simulink model "cic_filter_test"  (Simulink 7.4)
settings: Solver=ode45  StartTime=0.0  StopTime=100000  RelTol=1e-3
libraries: xbsIndex_r4 x178
(part 1 of 3)
settings Model: Creator=hong  LastModifiedBy=hong

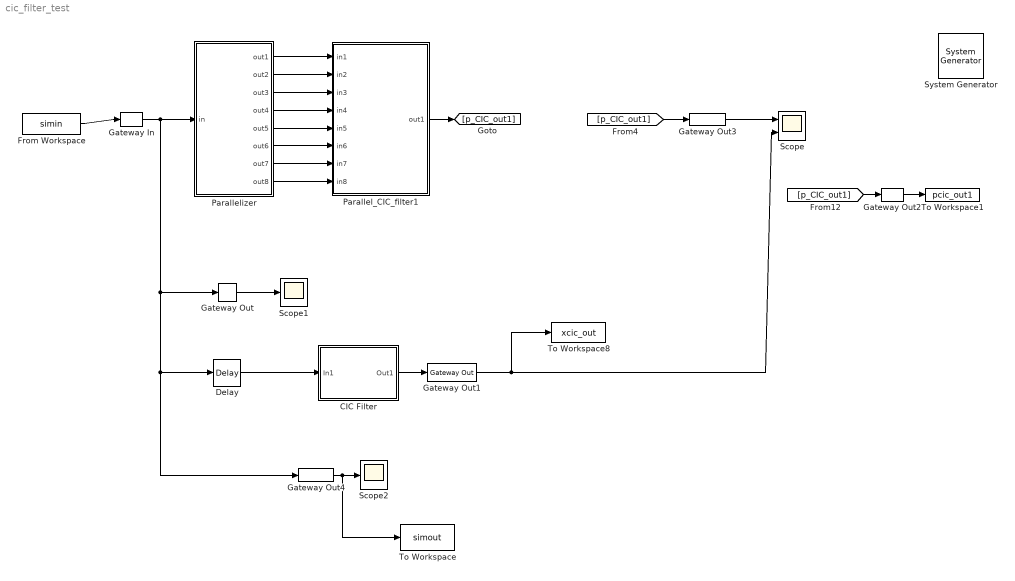
== system cic_filter_test ==
  " System Generator" : xbsIndex_r4/ System Generator  Tag=genX  SystemSampleTime=-1  xilinxfamily=virtex6  part=xc6vsx315t  speed=-3  package=ff1156  synthesis_tool=XST  clock_wrapper=Clock Enables  directory=./netlist  testbench=off  simulink_period=1  sysclk_period=10  dcm_input_clock_period=10  incr_netlist=off  trim_vbits=Everywhere in SubSystem  dbl_ovrd=According to Block Masks  core_generation=According to Block Masks  run_coregen=off  deprecated_control=off  eval_field=0  block_type=sysgen
      settings: block_version=11.4
  CIC Filter : Subsystem  mask(CIC Filter){input_bitwidth=8, input_binpt=7, filter_type=Decimator, rate_change=128, stages=3, m=1, pipeline=on}
      mask prompts: input_bitwidth "Input Bit Width"; input_binpt "Input Binary Point"; filter_type "Filter Type"; rate_change "Sample Rate Change"; stages "Number of Stages"; m "Differential Delay"; pipeline "Pipeline Differentiators"
      mask help: Cascaded Integrated Comb (CIC) Filter
      mask init:
      | % CIC Single Channel v1.0
      | % Set Block Logo
      | sav_gcb=gcb;
      | [bg,fg] = xlcmap('XBlock',0);
      | iPos = get_param(sav_gcb,'Position');
      | iWidth=iPos(3)-iPos(1); iHeight=iPos(4)-iPos(2);
      | iCx=iWidth/2;
      | iCy=iHeight/2;
      | [logoX, logoY] = xlogo(iPos);
      | 
      | % Determine previous filter type and number of stages
      | prev_stages_list = find_system(sav_gcb, 'lookUnderMasks', 'all', 'FollowLinks', 'on', 'Regexp', 'on', 'Name', '^Integrator*'); %this is a cell array
      | prev_stages = length(prev_stages_list);
      | 
      | prev_filter_list = find_system(sav_gcb, 'lookUnderMasks', 'all', 'FollowLinks', 'on', 'Regexp', 'on', 'Name', '^Up Sample*'); %this is a cell array
      | if (isempty(prev_filter_list))
      |     prev_filter_list = find_system(sav_gcb, 'lookUnderMasks', 'all', 'FollowLinks', 'on', 'Regexp', 'on', 'Name', '^Down Sample*'); %this is a cell array
      |     if (isempty(prev_filter_list))
      |         errordlg('Previous Filter Type could not be determined')
      |     else
      |         prev_filter_type = 2;
      |     end
      | else
      |     prev_filter_type = 1;
      | end
      |   
      |   
      | % Print label on the block
      | if(filter_type == 2)
      |    cic_str = sprintf('%d-Stage\n CIC\n%d:1 Decimator',stages, rate_change);
      | else
      |    cic_str = sprintf('%d-Stage\n CIC\n1:%d Interpolator',stages, rate_change);	
      | end
      | 
      | % Make sure the entered values for stages and channels are positive integers
      | nstages = round(sum(abs(stages)));
      | 
      | % issue an error if the number of stages entered is zero
      | if (nstages == 0)
      | 	nstages = prev_stages;
      | 	errordlg('Number of Stages must be more than zero')
      | end
      | 
      | if (nstages == prev_stages) & (filter_type == prev_filter_type)
      |     return
      | end
      | 
      | if(filter_type == 2) % Decimator
      |    if (prev_filter_type == 1) % was interpolator so turn to decimator
      |        for i= 2:prev_stages,
      | 	      delete_line(sav_gcb, ['Integrator' int2str(i-1) '/' int2str(1)], ['Integrator' int2str(i) '/' int2str(1)]);
      | 	      delete_line(sav_gcb, ['Differentiator' int2str(i-1) '/' int2str(1)], ['Differentiator' int2str(i) '/' int2str(1)]);
      |        end
      | 
      |        % disconnect the last blocks in the two sections
      |        delete_line(sav_gcb, ['Differentiator' int2str(prev_stages) '/' int2str(1)], ['Up Sample/1']);
      |        delete_line(sav_gcb, ['Integrator' int2str(prev_stages) '/' int2str(1)], 'Out1/1');
      | 	
      | 	   % delete the line from the Up sampler to the Integrator
      | 	   delete_line(sav_gcb, 'Up Sample/1', 'Integrator1/1'); 
      | 	   delete_line(sav_gcb, 'In1/1', 'Differentiator1/1'); 
      | 	   
      | 	   % Delete the Up Sampler and then replace with an Down Sampler
      | 	   pup = get_param([sav_gcb '/Up Sample'], 'position');
      | 	   delete_block([sav_gcb '/Up Sample']);
      | 	   load_system('xbsIndex_r4');
      | 	   add_block('xbsIndex_r4/Down Sample', [sav_gcb '/Down Sample'], 'sample_ratio', 'rate_change','sample_phase', 'First Value of Frame', 'position', [pup(1), pup(2), pup(3),pup(4)]);
      | 	   
      | 	   % Switch the Integrators and Decimators around
      | 	   for i=1:prev_stages,
      | 		   tempi = get_param([sav_gcb '/Integrator' int2str(i)], 'position');
      | 	       tempd = get_param([sav_gcb '/Differentiator' int2str(i)], 'position');
      | 		   set_param([sav_gcb '/Differentiator' int2str(i)], 'position', [tempi(1), tempi(2), tempi(3), tempi(4)], 'output_bitwidth', 'ceil(stages*log2(rate_change*m) + input_bitwidth)');
      | 		   set_param([sav_gcb '/Integrator' int2str(i)], 'position', [tempd(1), tempd(2), tempd(3), tempd(4)]);
      | 	   end
      | 	   	   	
      | 	   % add back in the lines
      |        add_line(sav_gcb, 'In1/1', 'Integrator1/1', 'autorouting', 'on');
      | 	   add_line(sav_gcb, ['Integrator' int2str(prev_stages) '/1'], 'Down Sample/1', 'autorouting', 'on');
      | 	   add_line(sav_gcb, 'Down Sample/1', 'Differentiator1/1', 'autorouting', 'on');
      | 	   add_line(sav_gcb, ['Differentiator' int2str(prev_stages) '/1'], 'Out1/1', 'autorouting', 'on');
      | 	   for i= 2:prev_stages,
      |           add_line(sav_gcb, ['Integrator' int2str(i-1) '/1'], ['Integrator' int2str(i) '/' int2str(1)], 'autorouting', 'on');
      |           add_line(sav_gcb, ['Differentiator' int2str(i-1) '/1'], ['Differentiator' int2str(i) '/' int2str(1)], 'autorouting', 'on');
      | 	   end
      | 		
      |        %Set the Output bit widths of Differentiator and Integrator stages
      |        set_param([sav_gcb '/Differentiator1'], 'output_bitwidth', 'ceil(stages*log2(rate_change*m) + input_bitwidth)');
      | 	   	   %Set the Output bit width of Integrator stages
      | 	   %Calculate the Interpolator Integrator Output Bit Growth
      |        for i= 1:prev_stages,
      | 			 j = nstages+i;
      | 	         set_param([sav_gcb '/Integrator' int2str(i)], 'output_bitwidth', 'ceil(stages*log2(rate_change*m) + input_bitwidth)');
      |              set_param([sav_gcb '/Differentiator' int2str(i)], 'output_bitwidth', 'ceil(stages*log2(rate_change*m) + input_bitwidth)');
      | 	   end
      | 	   
      |    end
      |    
      |    if (nstages ~= prev_stages)
      |     
      |        % disconnect all the wires from all the blocks
      |        for i= 2:prev_stages,
      | 	      delete_line(sav_gcb, ['Integrator' int2str(i-1) '/' int2str(1)], ['Integrator' int2str(i) '/' int2str(1)]);
      | 	      delete_line(sav_gcb, ['Differentiator' int2str(i-1) '/' int2str(1)], ['Differentiator' int2str(i) '/' int2str(1)]);
      |        end
      | 
      |        % disconnect the last blocks in the two sections
      |        delete_line(sav_gcb, ['Integrator' int2str(prev_stages) '/' int2str(1)], ['Down Sample/1']);
      |        delete_line(sav_gcb, ['Differentiator' int2str(prev_stages) '/' int2str(1)], 'Out1/1');
      | 	
      | 	   % delete the line from the down sampler to the differentiator
      | 	   delete_line(sav_gcb, 'Down Sample/1', 'Differentiator1/1');
      | 	
      | 	   % Remove all the blocks except the first one (as we always will have one)
      |        for i=2:prev_stages,
      | 		  delete_block([sav_gcb '/Differentiator' int2str(i)]);
      | 	      delete_block([sav_gcb '/Integrator' int2str(i)]);
      |        end
      | 	   
      | 	   %Set the Output bit width of Differentiator stages
      |        set_param([sav_gcb '/Differentiator1'], 'output_bitwidth', 'ceil(stages*log2(rate_change*m) + input_bitwidth)');
      | 	   
      | 	   % collect data on the position of existing blocks
      | 	   pi = get_param([sav_gcb '/Integrator1'], 'position');
      | 	   pd = get_param([sav_gcb '/Differentiator1'], 'position');
      | 	   set_param([sav_gcb '/Differentiator1'], 'position', [pi(1)+(nstages+1)*80, pd(2), pi(3)+(nstages+1)*80, pd(4)]);
      | 	   pd = get_param([sav_gcb '/Differentiator1'], 'position');
      | 	
      | 	   % move the current blocks to accomadate for new blocks to be added 
      | 	   pds = get_param([sav_gcb '/Down Sample'], 'position');
      | 	   set_param([sav_gcb '/Down Sample'], 'position', [pi(1)+(nstages)*80, pds(2), pi(3)+(nstages)*80, pds(4)]);
      | 	   
      | 	   po = get_param([sav_gcb '/Out1'], 'position');
      | 	   set_param([sav_gcb '/Out1'], 'position', [pd(1)+(nstages+1)*80, po(2), pd(1)+(po(3)-po(1))+(nstages+1)*80, po(4)]);	
      | 	
      | 	   % add back in the line between the Down Sampler and the 1st Differentiator
      |        add_line(sav_gcb, 'Down Sample/1', ['Differentiator1/' int2str(1)], 'autorouting', 'on');
      | 
      | 	   % Only add blocks if more than one stage is required
      | 	   if (nstages ~= 1)
      | 		
      | 	       % Add in a copy of the first block to make up the required number of stages
      |            for i=2:nstages,
      |                add_block([sav_gcb '/Integrator1'], [sav_gcb '/Integrator' int2str(i)], 'position', [pi(1)+(i-1)*80, pi(2), pi(3)+(i-1)*80, pi(4)]);
      | 		       add_block([sav_gcb '/Differentiator1'], [sav_gcb '/Differentiator' int2str(i)], 'position', [pd(1)+(i-1)*80, pd(2), pd(3)+(i-1)*80, pd(4)]);
      | 	       end
      | 		
      | 	       % Connect up the wires to each block use autorouting
      |            for i= 2:nstages,
      |  		       add_line(sav_gcb, ['Integrator' int2str(i-1) '/' int2str(1)], ['Integrator' int2str(i) '/' int2str(1)], 'autorouting', 'on');
      | 	           add_line(sav_gcb, ['Differentiator' int2str(i-1) '/' int2str(1)], ['Differentiator' int2str(i) '/' int2str(1)], 'autorouting', 'on');
      |            end
      | 	    end
      | 	       % Connect the last blocks in the two sections
      |            add_line(sav_gcb, ['Integrator' int2str(nstages) '/' int2str(1)], ['Down Sample/1'], 'autorouting', 'on');
      |            add_line(sav_gcb, ['Differentiator' int2str(nstages) '/' int2str(1)], ['Out1/1'], 'autorouting', 'on');
      |    end
      | 
      | else % Interpolator
      |    
      | 	
      | 	if (prev_filter_type == 2) % was decimator so turn to interpolator
      | 	
      | 	  % disconnect all the wires from all the blocks
      |        for i= 2:prev_stages,
      | 	      delete_line(sav_gcb, ['Integrator' int2str(i-1) '/' int2str(1)], ['Integrator' int2str(i) '/' int2str(1)]);
      | 	      delete_line(sav_gcb, ['Differentiator' int2str(i-1) '/' int2str(1)], ['Differentiator' int2str(i) '/' int2str(1)]);
      |        end
      | 
      |        % disconnect the last blocks in the two sections
      |        delete_line(sav_gcb, ['Integrator' int2str(prev_stages) '/' int2str(1)], ['Down Sample/1']);
      |        delete_line(sav_gcb, ['Differentiator' int2str(prev_stages) '/' int2str(1)], 'Out1/1');
      | 	
      | 	   % delete the line from the down sampler to the Differentiator
      | 	   delete_line(sav_gcb, 'Down Sample/1', 'Differentiator1/1'); 
      | 	   delete_line(sav_gcb, 'In1/1', 'Integrator1/1'); 
      | 	   
      | 	   % Delete the Down Sampler and then replace with a Up Sampler
      | 	   pdwn = get_param([sav_gcb '/Down Sample'], 'position');
      | 	   delete_block([sav_gcb '/Down Sample']);
      | 	   load_system('xbsIndex_r4');
      | 	   add_block('xbsIndex_r4/Up Sample', [sav_gcb '/Up Sample'], 'sample_ratio', 'rate_change', 'position', [pdwn(1), pdwn(2), pdwn(3), pdwn(4)]);
      | 	   
      | 	   % Switch the Integrators and Decimators around
      | 	   for i=1:prev_stages,
      | 		   tempi = get_param([sav_gcb '/Integrator' int2str(i)], 'position');
      | 	       tempd = get_param([sav_gcb '/Differentiator' int2str(i)], 'position');
      | 		   set_param([sav_gcb '/Differentiator' int2str(i)], 'position', [tempi(1), tempi(2), tempi(3), tempi(4)], 'output_bitwidth', [int2str(i) '+ input_bitwidth']);
      | 		   set_param([sav_gcb '/Integrator' int2str(i)], 'position', [tempd(1), tempd(2), tempd(3), tempd(4)]);
      | 	   end
      | 	   	   	
      | 	   % add back in the lines
      |        add_line(sav_gcb, 'In1/1', 'Differentiator1/1', 'autorouting', 'on');
      | 	   add_line(sav_gcb, ['Differentiator' int2str(prev_stages) '/1'], 'Up Sample/1', 'autorouting', 'on');
      | 	   add_line(sav_gcb, 'Up Sample/1', 'Integrator1/1', 'autorouting', 'on');
      | 	   add_line(sav_gcb, ['Integrator' int2str(prev_stages) '/1'], 'Out1/1', 'autorouting', 'on');
      | 	   for i= 2:prev_stages,
      |           add_line(sav_gcb, ['Integrator' int2str(i-1) '/1'], ['Integrator' int2str(i) '/1'], 'autorouting', 'on');
      |           add_line(sav_gcb, ['Differentiator' int2str(i-1) '/1'], ['Differentiator' int2str(i) '/1'], 'autorouting', 'on');
      | 	   end
      | 	   
      | 	   %Set the Output bit width of Integrator stages
      | 	   %Calculate the Interpolator Integrator Output Bit Growth
      |        for i= 1:prev_stages,
      | 			 j = nstages+i;
      | 	         set_param([sav_gcb '/Integrator' int2str(i)], 'output_bitwidth', ['ceil(log2(2^(2*stages-' int2str(j) ')*(rate_change*m)^(' int2str(j) '-stages)) + input_bitwidth)']);
      | 	   end
      | 		
      |    end
      |    
      | 	
      | 	if (nstages ~= prev_stages)
      |     
      |        % disconnect all the wires from all the blocks
      |        for i= 2:prev_stages,
      | 	      delete_line(sav_gcb, ['Integrator' int2str(i-1) '/' int2str(1)], ['Integrator' int2str(i) '/' int2str(1)]);
      | 	      delete_line(sav_gcb, ['Differentiator' int2str(i-1) '/' int2str(1)], ['Differentiator' int2str(i) '/' int2str(1)]);
      |        end
      | 
      |        % disconnect the last blocks in the two sections
      |        delete_line(sav_gcb, ['Differentiator' int2str(prev_stages) '/' int2str(1)], ['Up Sample/1']);
      |        delete_line(sav_gcb, ['Integrator' int2str(prev_stages) '/' int2str(1)], 'Out1/1');
      |        
      | 	
      | 	   % delete the line from the Up sampler to the Integrator1 for movement later
      | 	   delete_line(sav_gcb, 'Up Sample/1', 'Integrator1/1'); 
      | 	
      | 	   % Remove all the blocks except the first one (as we always will have one)
      |        for i=2:prev_stages,
      | 		  delete_block([sav_gcb '/Differentiator' int2str(i)]);
      | 	      delete_block([sav_gcb '/Integrator' int2str(i)]);
      |        end
      | 	
      | 	   %Set the Output bit width of first Differentiator stage (other are set as copies of this block)
      |        set_param([sav_gcb '/Differentiator1'], 'output_bitwidth', '1 + input_bitwidth');
      | 	   
      | 	   % collect data on the position of existing blocks
      | 	   pi = get_param([sav_gcb '/Integrator1'], 'position');
      | 	   pd = get_param([sav_gcb '/Differentiator1'], 'position');
      | 	   set_param([sav_gcb '/Integrator1'], 'position', [pd(1)+(nstages+1)*80, pi(2), pd(3)+(nstages+1)*80, pi(4)]);
      | 	   pi = get_param([sav_gcb '/Integrator1'], 'position');
      | 	
      | 	   % move the current blocks to accomadate for new blocks to be added 
      | 	   pus = get_param([sav_gcb '/Up Sample'], 'position');
      | 	   set_param([sav_gcb '/Up Sample'], 'position', [pd(1)+(nstages)*80, pus(2), pd(3)+(nstages)*80, pus(4)]);
      | 	
      | 	   po = get_param([sav_gcb '/Out1'], 'position');
      |        set_param([sav_gcb '/Out1'], 'position', [pi(1)+(nstages+1)*80, po(2), pi(1)+(po(3)-po(1))+(nstages+1)*80, po(4)]);	
      |       
      | 	
      | 	   % add back in the line between the Up Sampler and the 1st Integrator1
      | 	   add_line(sav_gcb, 'Up Sample/1', 'Integrator1/1', 'autorouting', 'on');
      | 	   
      | 	   % Only add blocks if more than one stage is required
      | 	   if (nstages ~= 1)
      | 		
      | 	       % Add in a copy of the first block to make up the required number of stages
      |            for i=2:nstages,
      |                add_block([sav_gcb '/Integrator1'], [sav_gcb '/Integrator' int2str(i)], 'position', [pi(1)+(i-1)*80, pi(2), pi(3)+(i-1)*80, pi(4)]);
      | 		       add_block([sav_gcb '/Differentiator1'], [sav_gcb '/Differentiator' int2str(i)], 'position', [pd(1)+(i-1)*80, pd(2), pd(3)+(i-1)*80, pd(4)], 'output_bitwidth', [int2str(i) '+ input_bitwidth']);
      | 	       end
      | 		
      | 	       % Connect up the wires to each block use autorouting
      |            for i= 2:nstages,
      |  		       add_line(sav_gcb, ['Integrator' int2str(i-1) '/' int2str(1)], ['Integrator' int2str(i) '/' int2str(1)], 'autorouting', 'on');
      | 	           add_line(sav_gcb, ['Differentiator' int2str(i-1) '/' int2str(1)], ['Differentiator' int2str(i) '/' int2str(1)], 'autorouting', 'on');
      |            end
      | 	    end
      | 	       % Connect the last blocks in the two sections
      |            add_line(sav_gcb, ['Differentiator' int2str(nstages) '/1'], ['Up Sample/1'], 'autorouting', 'on');
      |            add_line(sav_gcb, ['Integrator' int2str(nstages) '/1'], ['Out1/1'], 'autorouting', 'on');
      | 		   
      | 	     %Set the Output bit width of Integrator stages
      | 	     %Calculate the Interpolator Integrator Output Bit Growth
      |           for i= 1:nstages,
      | 			 j = nstages+i;
      | 	         set_param([sav_gcb '/Integrator' int2str(i)], 'output_bitwidth', ['ceil(log2(2^(2*stages-' int2str(j) ')*(rate_change*m)^(' int2str(j) '-stages)) + input_bitwidth)']);
      | 	      end
      |    end
      | 	  
      | end
      | 
      | 
      | % Set the pipelining to ON or OFF on the differentiators
      | if (pipeline == 0)
      | 	for i= 1:nstages
      | 		set_param([sav_gcb '/Differentiator' int2str(i), '/AddSub'], 'latency', '0')
      | 	end
      | else
      | 	for i= 1:nstages
      | 		set_param([sav_gcb '/Differentiator' int2str(i), '/AddSub'], 'latency' ,'1')
      | 	end
      | end
      settings: CopyFcn=set_param(gcb, 'MaskSelfModifiable', 'on', 'LinkStatus', 'none');
      mask Help: eval('');xlDoc('-book','sysgen','-topic','CIC_Filter');
      mask StyleString: edit,edit,popup(Interpolator|Decimator),edit,edit,popup(1|2|3|4),checkbox
      mask Display:
      | patch([0 iWidth iWidth 0],[0 0 iHeight iHeight] , bg);
      | patch(logoX,logoY , fg);
      | plot([0 0 iWidth iWidth 0], [0 iHeight iHeight 0 0]);
      | disp(cic_str)
  Delay : xbsIndex_r4/Delay  en=off  latency=5  dbl_ovrd=off  reg_retiming=off  block_type=delay
      settings: block_version=11.4
  From Workspace : FromWorkspace  VariableName=simin  SampleTime=0.01  Interpolate=off  OutputAfterFinalValue=Setting to zero
  Gateway In : xbsIndex_r4/Gateway In  arith_type="Signed  (2's comp)"  n_bits=8  bin_pt=7  quantization="Round  (unbiased: +/- Inf)"  overflow=Saturate  period=1  dbl_ovrd=off  timing_constraint=None  locs_specified=off  LOCs={}  hdl_port=on  block_type=gatewayin
      settings: infoedit="Gateway in block.  Converts inputs of type Simulink integer, double and fixed point to  Xilinx fixed point type.<br><br>Hardware notes:  In hardware these blocks become top level input ports."  block_version=11.4
  Gateway Out{,1..4} (5 alike) : xbsIndex_r4/Gateway Out  hdl_port=on  timing_constraint=None  locs_specified=off  LOCs={}  block_type=gatewayout
      settings: infoedit="Gateway out block.  Converts Xilinx fixed point inputs into ouputs of type Simulink integer, double, or fixed point.<br><br>Hardware notes:  In hardware these blocks become top level output ports or are discarded, depending on how they are configured."  block_version=11.4
  Parallel_CIC_filter1 : Subsystem  AncestorBlock=gbt_library/Parallel_CIC_filter  mask(Parallel_CIC_filter){n_stages=3, dec_rate=128, input_clk_rate=8, n_inputs=8, polyphase=off, add_latency=1, n_bits=8, bin_pt=7, dec2_halfout=on, half2first=off, recursives=[0 0 0 0 0 0 0 0 0 0], reduced_crtc_path=off}
      mask prompts: n_stages "CIC filter Order"; dec_rate "Decimation rate"; input_clk_rate "Input Clock Rate"; n_inputs "Number of inputs"; polyphase "polyphase structure?(Effective only when n_inputs = 1 or n_inputs = dec_rate)"; add_latency "Add latency"; n_bits "Input bit width"; bin_pt "Binary point"; dec2_halfout "When dec_rate =2, half the number of outputs?"; half2first "Order of stages: Smaller prime factors first?"; recursives "Recursive structure for each prime-factor stage"; reduced_crtc_path "In recursive stages, invoke reduced critical path structure?"
      mask help:
      | A non-recursive CIC filter with parallel inputs.
      | Decimation rate is factored into prime numbers. Each implemented using a single stage.
      |
      | Expecting a 1-dimensional boolean vector for
      | choosing the recursive/nonrecursive structure of each prime-factor stage.
      | ([0 1 1 0] means [non-recursive recursive recursive non-recursive] stages.)
      |
      | For each stages:
      | Only supports decimation rate that is a prime number.
      | If dec_rate = 2, then we can choose n_outputs = 0.5*n_inputs(less resource)
      |     or n_outputs = n_inputs.
      | In other cases, n_outputs = n_inputs.
      | Polyphase structure available for stages of n_inputs is 1 or 2.
      mask init:
      | config.source = str2func('parallel_cic_filter_init_xblock');
      | config.toplevel = gcb;
      | config.depend = get_dependlist('parallel_cic_filter'); 
      | set_param(gcb,'LinkStatus','inactive');
      | xBlock(config, {config.toplevel,...
      |                 'n_stages',n_stages, ...
      |                 'dec_rate', dec_rate, ...
      |                 'input_clk_rate', input_clk_rate, ...
      |                 'n_inputs', n_inputs,...
      |                 'polyphase', polyphase,...
      |                 'add_latency',add_latency,...
      |                 'dec2_halfout', dec2_halfout, ...
      |                 'half2first', half2first,...
      |                 'n_bits', n_bits, ...
      |                 'bin_pt', bin_pt,...
      |                 'reduced_crtc_path', reduced_crtc_path, ...
      |                 'recursives', recursives} ...
      |                 );
      | disp('new block added');
      settings: AttributesFormatString=|
      | dec_rate = 128
      | Order = 3
  Parallelizer : Subsystem  AncestorBlock=xblocks_library_misc/Parallelizer  mask(Parallelizer){n_outputs=8, sample_period=1}
      mask prompts: sample_period "sample_period (Input)"
      mask help:
      | Parallelizer takes in a single stream and convert it into
      | parallel outputs.
      | Output sample rate is input_sample_rate/n_outputs.
      mask init:
      | config.source=str2func('parallelizer_init_xblock');
      | config.depend=get_dependlist('parallelizer');
      | config.toplevel=gcb;
      | set_param(gcb,'LinkStatus','inactive');
      | xBlock(config, {config.toplevel,...
      |     'n_outputs', n_outputs, ...
      |     'sample_period', sample_period});
      settings: AttributesFormatString=Sample Period = 1
  Scope : Scope  NumInputPorts=2
      settings: YMin=-5~-5  YMax=5~5
  Scope1 : Scope
  Scope2 : Scope
      settings: SaveName=ScopeData2
  To Workspace : ToWorkspace  VariableName=simout  SampleTime=-1  SaveFormat=Structure
  To Workspace1 : ToWorkspace  VariableName=pcic_out1  SampleTime=-1  SaveFormat=Structure
  To Workspace8 : ToWorkspace  VariableName=xcic_out  SampleTime=-1  SaveFormat=Structure
  wires:
  Gateway In/1 -> Parallelizer/1(in), Gateway Out/1, Delay/1, Gateway Out4/1
  Parallelizer/1(out1) -> Parallel_CIC_filter1/1(in1)
  Parallelizer/2(out2) -> Parallel_CIC_filter1/2(in2)
  Parallelizer/3(out3) -> Parallel_CIC_filter1/3(in3)
  Parallelizer/4(out4) -> Parallel_CIC_filter1/4(in4)
  Parallelizer/5(out5) -> Parallel_CIC_filter1/5(in5)
  Parallelizer/6(out6) -> Parallel_CIC_filter1/6(in6)
  Parallelizer/7(out7) -> Parallel_CIC_filter1/7(in7)
  Parallelizer/8(out8) -> Parallel_CIC_filter1/8(in8)
  Gateway Out/1 -> Scope1/1
  Gateway Out1/1 -> Scope/2, To Workspace8/1
  CIC Filter/1(Out1) -> Gateway Out1/1
  Delay/1 -> CIC Filter/1(In1)
  Parallel_CIC_filter1/1(out1) -> [p_CIC_out1]
  [p_CIC_out1] -> Gateway Out2/1
  Gateway Out2/1 -> To Workspace1/1
  [p_CIC_out1] -> Gateway Out3/1
  Gateway Out3/1 -> Scope/1
  From Workspace/1 -> Gateway In/1
  Gateway Out4/1 -> Scope2/1, To Workspace/1

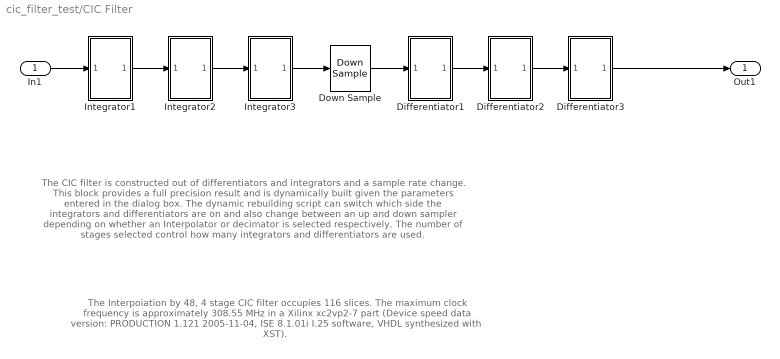
== system cic_filter_test/CIC Filter ==
  note: The CIC filter is constructed out of differentiators and integrators and
      | a sample rate change. This block provides a full precision result and is
      | dynamically built given the parameters entered in the dialog box. The
      | dynamic rebuilding script can switch which side the integrators and
      | differentiators are on and also change between an up and down sampler
      | depending on whether an Interpolator or decimator is selected respectively.
      | The number of stages selected control how many integrators and
      | differentiators are used.
  note: The Interpoiation by 48, 4 stage CIC filter occupies 116 slices.
      | The maximum clock frequency is approximately
      | 308.55 MHz in a Xilinx xc2vp2-7 part (Device speed data version:
      | PRODUCTION 1.121 2005-11-04, ISE 8.1.01i I.25 software, VHDL
      | synthesized with XST).
  In1 : Inport  OutDataType=sfix(16)  OutScaling=2^0
  Differentiator1 : Subsystem  mask(Differentiator Stage){m=m, output_bitwidth=ceil(stages*log2(rate_change*m) + input_bitwidth), output_binpt=input_binpt}
      mask prompts: m "Differential Delay"; output_bitwidth "Output Bit Width"; output_binpt "Output Binary Point"
      mask help: Multi-Channel Differentiator
      mask init:
      | set_param(gcb, 'LinkStatus', 'none');
  Differentiator2 : Subsystem  mask(Differentiator Stage){m=m, output_bitwidth=ceil(stages*log2(rate_change*m) + input_bitwidth), output_binpt=input_binpt}
      mask prompts: m "Differential Delay"; output_bitwidth "Output Bit Width"; output_binpt "Output Binary Point"
      mask help: Multi-Channel Differentiator
      mask init:
      | set_param(gcb, 'LinkStatus', 'none');
  Differentiator3 : Subsystem  mask(Differentiator Stage){m=m, output_bitwidth=ceil(stages*log2(rate_change*m) + input_bitwidth), output_binpt=input_binpt}
      mask prompts: m "Differential Delay"; output_bitwidth "Output Bit Width"; output_binpt "Output Binary Point"
      mask help: Multi-Channel Differentiator
      mask init:
      | set_param(gcb, 'LinkStatus', 'none');
  Down Sample : xbsIndex_r4/Down Sample  sample_ratio=rate_change  sample_phase=First Value of Frame  en=off  latency=1  dbl_ovrd=off  block_type=dsamp
      settings: block_version=9.2.00
  Integrator1 : Subsystem  mask(Integrator Stage){output_bitwidth=ceil(stages*log2(rate_change*m) + input_bitwidth)}
      mask prompts: output_bitwidth "Output Bit Width"
      mask help: Multi Channel Integrator
      mask init:
      | set_param(gcb, 'LinkStatus', 'none');
      settings: CopyFcn=set_param(gcb, 'LinkStatus', 'none');
  Integrator2 : Subsystem  mask(Integrator Stage){output_bitwidth=ceil(stages*log2(rate_change*m) + input_bitwidth)}
      mask prompts: output_bitwidth "Output Bit Width"
      mask help: Multi Channel Integrator
      mask init:
      | set_param(gcb, 'LinkStatus', 'none');
      settings: CopyFcn=set_param(gcb, 'LinkStatus', 'none');
  Integrator3 : Subsystem  mask(Integrator Stage){output_bitwidth=ceil(stages*log2(rate_change*m) + input_bitwidth)}
      mask prompts: output_bitwidth "Output Bit Width"
      mask help: Multi Channel Integrator
      mask init:
      | set_param(gcb, 'LinkStatus', 'none');
      settings: CopyFcn=set_param(gcb, 'LinkStatus', 'none');
  Out1 : Outport  OutDataType=sfix(16)  OutScaling=2^0
  wires:
  In1/1 -> Integrator1/1(In1)
  Down Sample/1 -> Differentiator1/1(In1)
  Integrator1/1(Out1) -> Integrator2/1(In1)
  Differentiator1/1(Out1) -> Differentiator2/1(In1)
  Integrator2/1(Out1) -> Integrator3/1(In1)
  Differentiator2/1(Out1) -> Differentiator3/1(In1)
  Integrator3/1(Out1) -> Down Sample/1
  Differentiator3/1(Out1) -> Out1/1

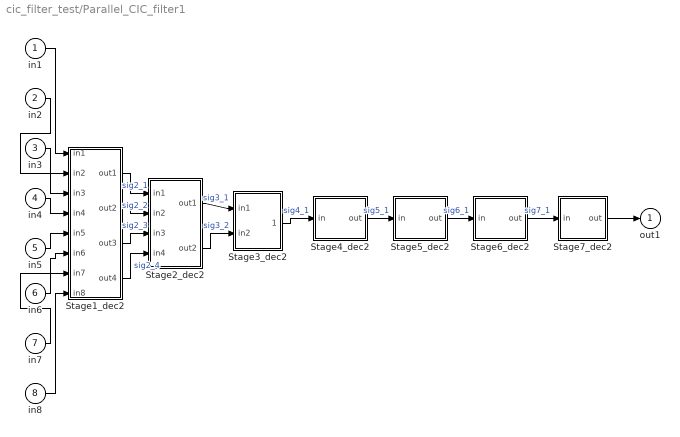
== system cic_filter_test/Parallel_CIC_filter1 ==
  in1 : Inport
  in2 : Inport  Port=2
  in3 : Inport  Port=3
  in4 : Inport  Port=4
  in5 : Inport  Port=5
  in6 : Inport  Port=6
  in7 : Inport  Port=7
  in8 : Inport  Port=8
  Stage1_dec2 : Subsystem
      settings: AttributesFormatString=|
      | nonrecursive
      | 8_in
      | polyphase:off
  Stage2_dec2 : Subsystem
      settings: AttributesFormatString=|
      | nonrecursive
      | 11_in
      | polyphase:off
  Stage3_dec2 : Subsystem
      settings: AttributesFormatString=|
      | nonrecursive
      | 14_in
      | polyphase:off
  Stage4_dec2 : Subsystem
      settings: AttributesFormatString=|
      | nonrecursive
      | 17_in
      | polyphase:off
  Stage5_dec2 : Subsystem
      settings: AttributesFormatString=|
      | nonrecursive
      | 20_in
      | polyphase:off
  Stage6_dec2 : Subsystem
      settings: AttributesFormatString=|
      | nonrecursive
      | 23_in
      | polyphase:off
  Stage7_dec2 : Subsystem
      settings: AttributesFormatString=|
      | nonrecursive
      | 26_in
      | polyphase:off
  out1 : Outport
  wires:
  Stage7_dec2/1(out) -> out1/1
  Stage6_dec2/1(out) -> Stage7_dec2/1(in)  "sig7_1"
  Stage5_dec2/1(out) -> Stage6_dec2/1(in)  "sig6_1"
  Stage4_dec2/1(out) -> Stage5_dec2/1(in)  "sig5_1"
  Stage3_dec2/1(out1) -> Stage4_dec2/1(in)  "sig4_1"
  Stage2_dec2/2(out2) -> Stage3_dec2/2(in2)  "sig3_2"
  Stage2_dec2/1(out1) -> Stage3_dec2/1(in1)  "sig3_1"
  Stage1_dec2/4(out4) -> Stage2_dec2/4(in4)  "sig2_4"
  Stage1_dec2/3(out3) -> Stage2_dec2/3(in3)  "sig2_3"
  Stage1_dec2/2(out2) -> Stage2_dec2/2(in2)  "sig2_2"
  Stage1_dec2/1(out1) -> Stage2_dec2/1(in1)  "sig2_1"
  in8/1 -> Stage1_dec2/8(in8)
  in7/1 -> Stage1_dec2/7(in7)
  in6/1 -> Stage1_dec2/6(in6)
  in5/1 -> Stage1_dec2/5(in5)
  in4/1 -> Stage1_dec2/4(in4)
  in3/1 -> Stage1_dec2/3(in3)
  in2/1 -> Stage1_dec2/2(in2)
  in1/1 -> Stage1_dec2/1(in1)

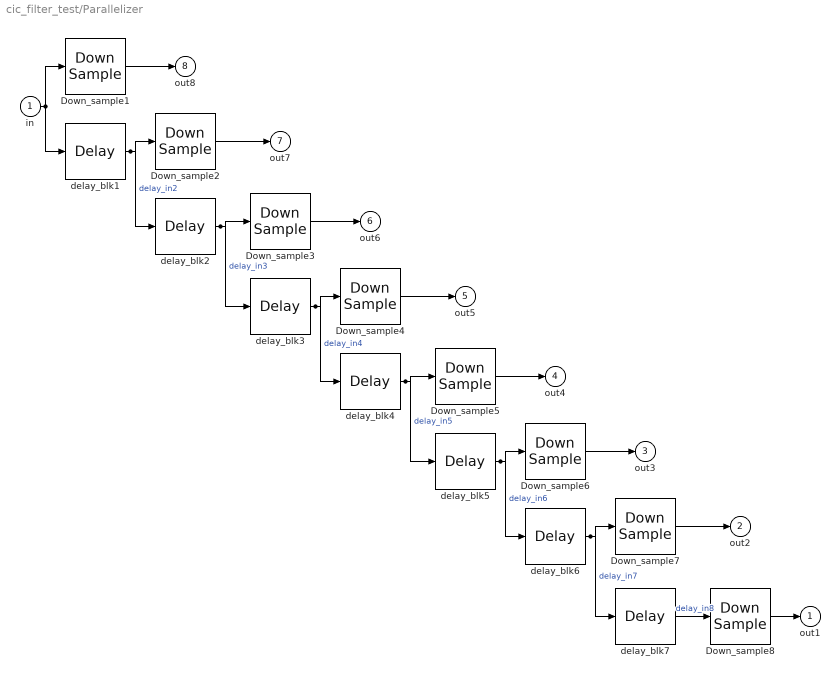
== system cic_filter_test/Parallelizer ==
  in : Inport
  Down_sample{1..8} (8 alike) : xbsIndex_r4/Down Sample  sample_ratio=8  sample_phase="Last Value of Frame  (most efficient)"  en=off  latency=1  dbl_ovrd=off  block_type=dsamp
      settings: block_version=11.4
  delay_blk{1..7} (7 alike) : xbsIndex_r4/Delay  en=off  latency=1  dbl_ovrd=off  reg_retiming=off  block_type=delay
      settings: block_version=11.4
  out1 : Outport
  out2 : Outport  Port=2
  out3 : Outport  Port=3
  out4 : Outport  Port=4
  out5 : Outport  Port=5
  out6 : Outport  Port=6
  out7 : Outport  Port=7
  out8 : Outport  Port=8
  wires:
  in/1 -> Down_sample1/1, delay_blk1/1
  delay_blk1/1 -> Down_sample2/1, delay_blk2/1  "delay_in2"
  delay_blk2/1 -> Down_sample3/1, delay_blk3/1  "delay_in3"
  delay_blk3/1 -> Down_sample4/1, delay_blk4/1  "delay_in4"
  delay_blk4/1 -> Down_sample5/1, delay_blk5/1  "delay_in5"
  delay_blk5/1 -> Down_sample6/1, delay_blk6/1  "delay_in6"
  delay_blk6/1 -> Down_sample7/1, delay_blk7/1  "delay_in7"
  Down_sample8/1 -> out1/1
  delay_blk7/1 -> Down_sample8/1  "delay_in8"
  Down_sample7/1 -> out2/1
  Down_sample6/1 -> out3/1
  Down_sample5/1 -> out4/1
  Down_sample4/1 -> out5/1
  Down_sample3/1 -> out6/1
  Down_sample2/1 -> out7/1
  Down_sample1/1 -> out8/1

== system cic_filter_test/CIC Filter/Differentiator1 ==
  In1 : Inport  OutDataType=sfix(16)  OutScaling=2^0
  AddSub : xbsIndex_r4/AddSub  mode=Subtraction  use_carryin=off  use_carryout=off  en=off  latency=1  precision=User Defined  arith_type="Signed  (2's comp)"  n_bits=output_bitwidth  bin_pt=output_binpt  quantization=Truncate  overflow=Wrap  dbl_ovrd=off  use_behavioral_HDL=on  hw_selection=Fabric  pipelined=off  use_rpm=on  block_type=addsub
      settings: xl_area=[53 106 0 106 0 0 0]  block_version=VER_STRING_GOES_HERE
  Delay : xbsIndex_r4/Delay  en=off  latency=m  dbl_ovrd=off  reg_retiming=off  block_type=delay
      settings: infoedit="Delay line having  configurable length.<P><P>Hardware notes: A delay line is a chain, each link of which is an SRL16 followed by a flip-flop. If register retiming is enabled, the delay line is a chain of flip-flops."  xl_area=[53 106 0 0 0 0 0]  block_version=VER_STRING_GOES_HERE
  Out1 : Outport  OutDataType=sfix(16)  OutScaling=2^0
  wires:
  In1/1 -> Delay/1, AddSub/1
  AddSub/1 -> Out1/1
  Delay/1 -> AddSub/2

== system cic_filter_test/CIC Filter/Differentiator2 ==
  In1 : Inport  OutDataType=sfix(16)  OutScaling=2^0
  AddSub : xbsIndex_r4/AddSub  mode=Subtraction  use_carryin=off  use_carryout=off  en=off  latency=1  precision=User Defined  arith_type="Signed  (2's comp)"  n_bits=output_bitwidth  bin_pt=output_binpt  quantization=Truncate  overflow=Wrap  dbl_ovrd=off  use_behavioral_HDL=on  hw_selection=Fabric  pipelined=off  use_rpm=on  block_type=addsub
      settings: xl_area=[53 106 0 106 0 0 0]  block_version=VER_STRING_GOES_HERE
  Delay : xbsIndex_r4/Delay  en=off  latency=m  dbl_ovrd=off  reg_retiming=off  block_type=delay
      settings: infoedit="Delay line having  configurable length.<P><P>Hardware notes: A delay line is a chain, each link of which is an SRL16 followed by a flip-flop. If register retiming is enabled, the delay line is a chain of flip-flops."  xl_area=[53 106 0 0 0 0 0]  block_version=VER_STRING_GOES_HERE
  Out1 : Outport  OutDataType=sfix(16)  OutScaling=2^0
  wires:
  Delay/1 -> AddSub/2
  AddSub/1 -> Out1/1
  In1/1 -> AddSub/1, Delay/1

== system cic_filter_test/CIC Filter/Differentiator3 ==
  In1 : Inport  OutDataType=sfix(16)  OutScaling=2^0
  AddSub : xbsIndex_r4/AddSub  mode=Subtraction  use_carryin=off  use_carryout=off  en=off  latency=1  precision=User Defined  arith_type="Signed  (2's comp)"  n_bits=output_bitwidth  bin_pt=output_binpt  quantization=Truncate  overflow=Wrap  dbl_ovrd=off  use_behavioral_HDL=on  hw_selection=Fabric  pipelined=off  use_rpm=on  block_type=addsub
      settings: xl_area=[53 106 0 106 0 0 0]  block_version=VER_STRING_GOES_HERE
  Delay : xbsIndex_r4/Delay  en=off  latency=m  dbl_ovrd=off  reg_retiming=off  block_type=delay
      settings: infoedit="Delay line having  configurable length.<P><P>Hardware notes: A delay line is a chain, each link of which is an SRL16 followed by a flip-flop. If register retiming is enabled, the delay line is a chain of flip-flops."  xl_area=[53 106 0 0 0 0 0]  block_version=VER_STRING_GOES_HERE
  Out1 : Outport  OutDataType=sfix(16)  OutScaling=2^0
  wires:
  Delay/1 -> AddSub/2
  AddSub/1 -> Out1/1
  In1/1 -> AddSub/1, Delay/1

== system cic_filter_test/CIC Filter/Integrator1 ==
  In1 : Inport  OutDataType=sfix(16)  OutScaling=2^0
  Accumulator : xbsIndex_r4/Accumulator  operation=Add  n_bits=output_bitwidth  overflow=Wrap  scale=1  rst=off  hasbypass=off  en=off  dbl_ovrd=off  use_behavioral_HDL=on  implementation=Fabric  block_type=accum
      settings: infoedit="Adder or subtractor-based accumulator.   Output type and binary point position match the input.<P><P>Hardware notes: When \"Reinitialize with Input 'b' on Reset\" is selected, the accumulator is forced to run at the system rate even if the input 'b' is running at a slower rate."  xl_area=[53 106 0 106 0 0 0]  block_version=VER_STRING_GOES_HERE
  Out1 : Outport  OutDataType=sfix(16)  OutScaling=2^0
  wires:
  In1/1 -> Accumulator/1
  Accumulator/1 -> Out1/1

== system cic_filter_test/CIC Filter/Integrator2 ==
  In1 : Inport  OutDataType=sfix(16)  OutScaling=2^0
  Accumulator : xbsIndex_r4/Accumulator  operation=Add  n_bits=output_bitwidth  overflow=Wrap  scale=1  rst=off  hasbypass=off  en=off  dbl_ovrd=off  use_behavioral_HDL=on  implementation=Fabric  block_type=accum
      settings: infoedit="Adder or subtractor-based accumulator.   Output type and binary point position match the input.<P><P>Hardware notes: When \"Reinitialize with Input 'b' on Reset\" is selected, the accumulator is forced to run at the system rate even if the input 'b' is running at a slower rate."  xl_area=[53 106 0 106 0 0 0]  block_version=VER_STRING_GOES_HERE
  Out1 : Outport  OutDataType=sfix(16)  OutScaling=2^0
  wires:
  Accumulator/1 -> Out1/1
  In1/1 -> Accumulator/1

== system cic_filter_test/CIC Filter/Integrator3 ==
  In1 : Inport  OutDataType=sfix(16)  OutScaling=2^0
  Accumulator : xbsIndex_r4/Accumulator  operation=Add  n_bits=output_bitwidth  overflow=Wrap  scale=1  rst=off  hasbypass=off  en=off  dbl_ovrd=off  use_behavioral_HDL=on  implementation=Fabric  block_type=accum
      settings: infoedit="Adder or subtractor-based accumulator.   Output type and binary point position match the input.<P><P>Hardware notes: When \"Reinitialize with Input 'b' on Reset\" is selected, the accumulator is forced to run at the system rate even if the input 'b' is running at a slower rate."  xl_area=[53 106 0 106 0 0 0]  block_version=VER_STRING_GOES_HERE
  Out1 : Outport  OutDataType=sfix(16)  OutScaling=2^0
  wires:
  Accumulator/1 -> Out1/1
  In1/1 -> Accumulator/1

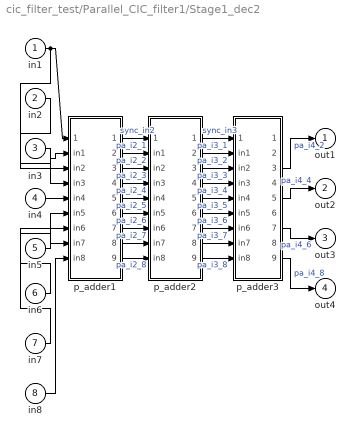
== system cic_filter_test/Parallel_CIC_filter1/Stage1_dec2 ==
  in1 : Inport
  in2 : Inport  Port=2
  in3 : Inport  Port=3
  in4 : Inport  Port=4
  in5 : Inport  Port=5
  in6 : Inport  Port=6
  in7 : Inport  Port=7
  in8 : Inport  Port=8
  p_adder1 : Subsystem
      settings: AttributesFormatString=|
      | Accumulation Length = 2
      | Add Latency = 1
      | Delay Length =1
  p_adder2 : Subsystem
      settings: AttributesFormatString=|
      | Accumulation Length = 2
      | Add Latency = 1
      | Delay Length =1
  p_adder3 : Subsystem
      settings: AttributesFormatString=|
      | Accumulation Length = 2
      | Add Latency = 1
      | Delay Length =1
  out1 : Outport
  out2 : Outport  Port=2
  out3 : Outport  Port=3
  out4 : Outport  Port=4
  wires:
  in1/1 -> p_adder1/2(in1), p_adder1/1(sync_in)
  p_adder3/9(out8) -> out4/1  "pa_i4_8"
  p_adder3/7(out6) -> out3/1  "pa_i4_6"
  p_adder3/5(out4) -> out2/1  "pa_i4_4"
  p_adder3/3(out2) -> out1/1  "pa_i4_2"
  p_adder2/9(out8) -> p_adder3/9(in8)  "pa_i3_8"
  p_adder2/8(out7) -> p_adder3/8(in7)  "pa_i3_7"
  p_adder2/7(out6) -> p_adder3/7(in6)  "pa_i3_6"
  p_adder2/6(out5) -> p_adder3/6(in5)  "pa_i3_5"
  p_adder2/5(out4) -> p_adder3/5(in4)  "pa_i3_4"
  p_adder2/4(out3) -> p_adder3/4(in3)  "pa_i3_3"
  p_adder2/3(out2) -> p_adder3/3(in2)  "pa_i3_2"
  p_adder2/2(out1) -> p_adder3/2(in1)  "pa_i3_1"
  p_adder2/1(sync_out) -> p_adder3/1(sync_in)  "sync_in3"
  p_adder1/9(out8) -> p_adder2/9(in8)  "pa_i2_8"
  p_adder1/8(out7) -> p_adder2/8(in7)  "pa_i2_7"
  p_adder1/7(out6) -> p_adder2/7(in6)  "pa_i2_6"
  p_adder1/6(out5) -> p_adder2/6(in5)  "pa_i2_5"
  p_adder1/5(out4) -> p_adder2/5(in4)  "pa_i2_4"
  p_adder1/4(out3) -> p_adder2/4(in3)  "pa_i2_3"
  p_adder1/3(out2) -> p_adder2/3(in2)  "pa_i2_2"
  p_adder1/2(out1) -> p_adder2/2(in1)  "pa_i2_1"
  p_adder1/1(sync_out) -> p_adder2/1(sync_in)  "sync_in2"
  in8/1 -> p_adder1/9(in8)
  in7/1 -> p_adder1/8(in7)
  in6/1 -> p_adder1/7(in6)
  in5/1 -> p_adder1/6(in5)
  in4/1 -> p_adder1/5(in4)
  in3/1 -> p_adder1/4(in3)
  in2/1 -> p_adder1/3(in2)

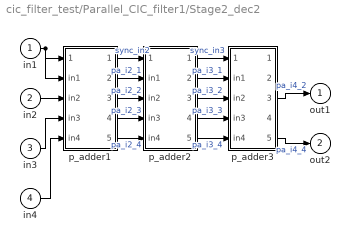
== system cic_filter_test/Parallel_CIC_filter1/Stage2_dec2 ==
  in1 : Inport
  in2 : Inport  Port=2
  in3 : Inport  Port=3
  in4 : Inport  Port=4
  p_adder1 : Subsystem
      settings: AttributesFormatString=|
      | Accumulation Length = 2
      | Add Latency = 1
      | Delay Length =1
  p_adder2 : Subsystem
      settings: AttributesFormatString=|
      | Accumulation Length = 2
      | Add Latency = 1
      | Delay Length =1
  p_adder3 : Subsystem
      settings: AttributesFormatString=|
      | Accumulation Length = 2
      | Add Latency = 1
      | Delay Length =1
  out1 : Outport
  out2 : Outport  Port=2
  wires:
  in1/1 -> p_adder1/2(in1), p_adder1/1(sync_in)
  p_adder3/5(out4) -> out2/1  "pa_i4_4"
  p_adder3/3(out2) -> out1/1  "pa_i4_2"
  p_adder2/5(out4) -> p_adder3/5(in4)  "pa_i3_4"
  p_adder2/4(out3) -> p_adder3/4(in3)  "pa_i3_3"
  p_adder2/3(out2) -> p_adder3/3(in2)  "pa_i3_2"
  p_adder2/2(out1) -> p_adder3/2(in1)  "pa_i3_1"
  p_adder2/1(sync_out) -> p_adder3/1(sync_in)  "sync_in3"
  p_adder1/5(out4) -> p_adder2/5(in4)  "pa_i2_4"
  p_adder1/4(out3) -> p_adder2/4(in3)  "pa_i2_3"
  p_adder1/3(out2) -> p_adder2/3(in2)  "pa_i2_2"
  p_adder1/2(out1) -> p_adder2/2(in1)  "pa_i2_1"
  p_adder1/1(sync_out) -> p_adder2/1(sync_in)  "sync_in2"
  in4/1 -> p_adder1/5(in4)
  in3/1 -> p_adder1/4(in3)
  in2/1 -> p_adder1/3(in2)

== system cic_filter_test/Parallel_CIC_filter1/Stage3_dec2 ==
  in1 : Inport
  in2 : Inport  Port=2
  p_adder1 : Subsystem
      settings: AttributesFormatString=|
      | Accumulation Length = 2
      | Add Latency = 1
      | Delay Length =1
  p_adder2 : Subsystem
      settings: AttributesFormatString=|
      | Accumulation Length = 2
      | Add Latency = 1
      | Delay Length =1
  p_adder3 : Subsystem
      settings: AttributesFormatString=|
      | Accumulation Length = 2
      | Add Latency = 1
      | Delay Length =1
  out1 : Outport
  wires:
  in1/1 -> p_adder1/2(in1), p_adder1/1(sync_in)
  p_adder3/3(out2) -> out1/1  "pa_i4_2"
  p_adder2/3(out2) -> p_adder3/3(in2)  "pa_i3_2"
  p_adder2/2(out1) -> p_adder3/2(in1)  "pa_i3_1"
  p_adder2/1(sync_out) -> p_adder3/1(sync_in)  "sync_in3"
  p_adder1/3(out2) -> p_adder2/3(in2)  "pa_i2_2"
  p_adder1/2(out1) -> p_adder2/2(in1)  "pa_i2_1"
  p_adder1/1(sync_out) -> p_adder2/1(sync_in)  "sync_in2"
  in2/1 -> p_adder1/3(in2)

== system cic_filter_test/Parallel_CIC_filter1/Stage4_dec2 ==
  in : Inport
  Down_sample1 : Subsystem
  adder_tree1 : Subsystem
  adder_tree2 : Subsystem
  adder_tree3 : Subsystem
  delay1_1 : xbsIndex_r4/Delay  en=off  latency=1  dbl_ovrd=off  reg_retiming=off  block_type=delay
      settings: block_version=11.4
  delay2_1 : xbsIndex_r4/Delay  en=off  latency=1  dbl_ovrd=off  reg_retiming=off  block_type=delay
      settings: block_version=11.4
  delay3_1 : xbsIndex_r4/Delay  en=off  latency=1  dbl_ovrd=off  reg_retiming=off  block_type=delay
      settings: block_version=11.4
  out : Outport
  wires:
  in/1 -> adder_tree1/2(din_1), adder_tree1/1(sync), delay1_1/1
  adder_tree1/2(dout) -> adder_tree2/2(din_1), delay2_1/1  "delay_in1_1"
  adder_tree2/2(dout) -> adder_tree3/2(din_1), delay3_1/1  "delay_in2_1"
  Down_sample1/1(Out) -> out/1
  adder_tree3/2(dout) -> Down_sample1/1(In)  "delay_in3_1"
  delay3_1/1 -> adder_tree3/3(din_2)  "delay_out3_2"
  adder_tree2/1(sync_out) -> adder_tree3/1(sync)  "adder_tree_sync_in3"
  delay2_1/1 -> adder_tree2/3(din_2)  "delay_out2_2"
  adder_tree1/1(sync_out) -> adder_tree2/1(sync)  "adder_tree_sync_in2"
  delay1_1/1 -> adder_tree1/3(din_2)  "delay_out1_2"

== system cic_filter_test/Parallel_CIC_filter1/Stage5_dec2 ==
  in : Inport
  Down_sample1 : Subsystem
  adder_tree1 : Subsystem
  adder_tree2 : Subsystem
  adder_tree3 : Subsystem
  delay1_1 : xbsIndex_r4/Delay  en=off  latency=2  dbl_ovrd=off  reg_retiming=off  block_type=delay
      settings: block_version=11.4
  delay2_1 : xbsIndex_r4/Delay  en=off  latency=2  dbl_ovrd=off  reg_retiming=off  block_type=delay
      settings: block_version=11.4
  delay3_1 : xbsIndex_r4/Delay  en=off  latency=2  dbl_ovrd=off  reg_retiming=off  block_type=delay
      settings: block_version=11.4
  out : Outport
  wires:
  in/1 -> adder_tree1/2(din_1), adder_tree1/1(sync), delay1_1/1
  adder_tree1/2(dout) -> adder_tree2/2(din_1), delay2_1/1  "delay_in1_1"
  adder_tree2/2(dout) -> adder_tree3/2(din_1), delay3_1/1  "delay_in2_1"
  Down_sample1/1(Out) -> out/1
  adder_tree3/2(dout) -> Down_sample1/1(In)  "delay_in3_1"
  delay3_1/1 -> adder_tree3/3(din_2)  "delay_out3_2"
  adder_tree2/1(sync_out) -> adder_tree3/1(sync)  "adder_tree_sync_in3"
  delay2_1/1 -> adder_tree2/3(din_2)  "delay_out2_2"
  adder_tree1/1(sync_out) -> adder_tree2/1(sync)  "adder_tree_sync_in2"
  delay1_1/1 -> adder_tree1/3(din_2)  "delay_out1_2"

== system cic_filter_test/Parallel_CIC_filter1/Stage6_dec2 ==
  in : Inport
  Down_sample1 : Subsystem
  adder_tree1 : Subsystem
  adder_tree2 : Subsystem
  adder_tree3 : Subsystem
  delay1_1 : xbsIndex_r4/Delay  en=off  latency=4  dbl_ovrd=off  reg_retiming=off  block_type=delay
      settings: block_version=11.4
  delay2_1 : xbsIndex_r4/Delay  en=off  latency=4  dbl_ovrd=off  reg_retiming=off  block_type=delay
      settings: block_version=11.4
  delay3_1 : xbsIndex_r4/Delay  en=off  latency=4  dbl_ovrd=off  reg_retiming=off  block_type=delay
      settings: block_version=11.4
  out : Outport
  wires:
  in/1 -> adder_tree1/2(din_1), adder_tree1/1(sync), delay1_1/1
  adder_tree1/2(dout) -> adder_tree2/2(din_1), delay2_1/1  "delay_in1_1"
  adder_tree2/2(dout) -> adder_tree3/2(din_1), delay3_1/1  "delay_in2_1"
  Down_sample1/1(Out) -> out/1
  adder_tree3/2(dout) -> Down_sample1/1(In)  "delay_in3_1"
  delay3_1/1 -> adder_tree3/3(din_2)  "delay_out3_2"
  adder_tree2/1(sync_out) -> adder_tree3/1(sync)  "adder_tree_sync_in3"
  delay2_1/1 -> adder_tree2/3(din_2)  "delay_out2_2"
  adder_tree1/1(sync_out) -> adder_tree2/1(sync)  "adder_tree_sync_in2"
  delay1_1/1 -> adder_tree1/3(din_2)  "delay_out1_2"

== system cic_filter_test/Parallel_CIC_filter1/Stage7_dec2 ==
  in : Inport
  Down_sample1 : Subsystem
  adder_tree1 : Subsystem
  adder_tree2 : Subsystem
  adder_tree3 : Subsystem
  delay1_1 : xbsIndex_r4/Delay  en=off  latency=8  dbl_ovrd=off  reg_retiming=off  block_type=delay
      settings: block_version=11.4
  delay2_1 : xbsIndex_r4/Delay  en=off  latency=8  dbl_ovrd=off  reg_retiming=off  block_type=delay
      settings: block_version=11.4
  delay3_1 : xbsIndex_r4/Delay  en=off  latency=8  dbl_ovrd=off  reg_retiming=off  block_type=delay
      settings: block_version=11.4
  out : Outport
  wires:
  in/1 -> adder_tree1/2(din_1), adder_tree1/1(sync), delay1_1/1
  adder_tree1/2(dout) -> adder_tree2/2(din_1), delay2_1/1  "delay_in1_1"
  adder_tree2/2(dout) -> adder_tree3/2(din_1), delay3_1/1  "delay_in2_1"
  Down_sample1/1(Out) -> out/1
  adder_tree3/2(dout) -> Down_sample1/1(In)  "delay_in3_1"
  delay3_1/1 -> adder_tree3/3(din_2)  "delay_out3_2"
  adder_tree2/1(sync_out) -> adder_tree3/1(sync)  "adder_tree_sync_in3"
  delay2_1/1 -> adder_tree2/3(din_2)  "delay_out2_2"
  adder_tree1/1(sync_out) -> adder_tree2/1(sync)  "adder_tree_sync_in2"
  delay1_1/1 -> adder_tree1/3(din_2)  "delay_out1_2"

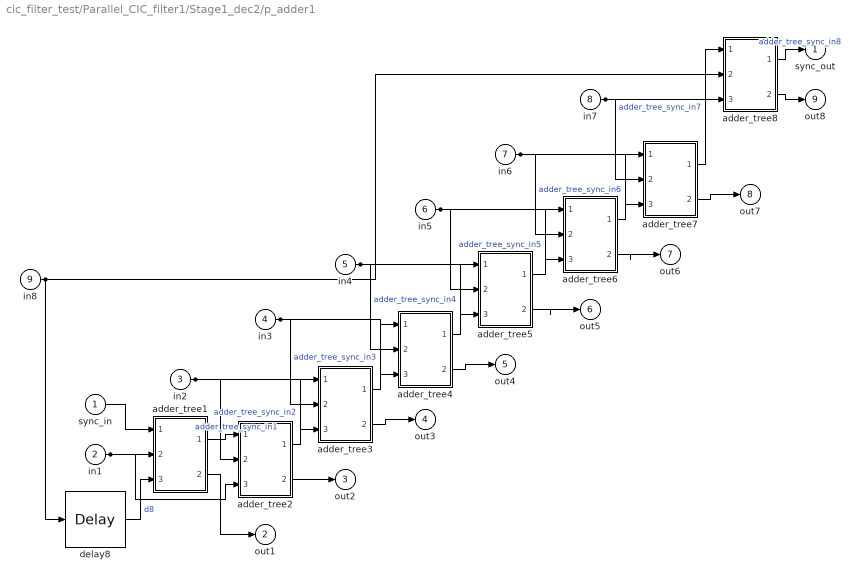
== system cic_filter_test/Parallel_CIC_filter1/Stage1_dec2/p_adder1 ==
  sync_in : Inport
  in1 : Inport  Port=2
  in2 : Inport  Port=3
  in3 : Inport  Port=4
  in4 : Inport  Port=5
  in5 : Inport  Port=6
  in6 : Inport  Port=7
  in7 : Inport  Port=8
  in8 : Inport  Port=9
  adder_tree1 : Subsystem
  adder_tree2 : Subsystem
  adder_tree3 : Subsystem
  adder_tree4 : Subsystem
  adder_tree5 : Subsystem
  adder_tree6 : Subsystem
  adder_tree7 : Subsystem
  adder_tree8 : Subsystem
  delay8 : xbsIndex_r4/Delay  en=off  latency=1  dbl_ovrd=off  reg_retiming=off  block_type=delay
      settings: block_version=11.4
  sync_out : Outport
  out1 : Outport  Port=2
  out2 : Outport  Port=3
  out3 : Outport  Port=4
  out4 : Outport  Port=5
  out5 : Outport  Port=6
  out6 : Outport  Port=7
  out7 : Outport  Port=8
  out8 : Outport  Port=9
  wires:
  in8/1 -> adder_tree8/2(din_1), delay8/1
  in1/1 -> adder_tree2/3(din_2), adder_tree1/2(din_1)
  in2/1 -> adder_tree3/3(din_2), adder_tree2/2(din_1)
  in3/1 -> adder_tree4/3(din_2), adder_tree3/2(din_1)
  in4/1 -> adder_tree5/3(din_2), adder_tree4/2(din_1)
  in5/1 -> adder_tree6/3(din_2), adder_tree5/2(din_1)
  in6/1 -> adder_tree7/3(din_2), adder_tree6/2(din_1)
  in7/1 -> adder_tree8/3(din_2), adder_tree7/2(din_1)
  adder_tree8/1(sync_out) -> sync_out/1  "adder_tree_sync_in8"
  adder_tree8/2(dout) -> out8/1
  adder_tree7/1(sync_out) -> adder_tree8/1(sync)  "adder_tree_sync_in7"
  adder_tree7/2(dout) -> out7/1
  adder_tree6/1(sync_out) -> adder_tree7/1(sync)  "adder_tree_sync_in6"
  adder_tree6/2(dout) -> out6/1
  adder_tree5/1(sync_out) -> adder_tree6/1(sync)  "adder_tree_sync_in5"
  adder_tree5/2(dout) -> out5/1
  adder_tree4/1(sync_out) -> adder_tree5/1(sync)  "adder_tree_sync_in4"
  adder_tree4/2(dout) -> out4/1
  adder_tree3/1(sync_out) -> adder_tree4/1(sync)  "adder_tree_sync_in3"
  adder_tree3/2(dout) -> out3/1
  adder_tree2/1(sync_out) -> adder_tree3/1(sync)  "adder_tree_sync_in2"
  adder_tree2/2(dout) -> out2/1
  adder_tree1/1(sync_out) -> adder_tree2/1(sync)  "adder_tree_sync_in1"
  adder_tree1/2(dout) -> out1/1
  delay8/1 -> adder_tree1/3(din_2)  "d8"
  sync_in/1 -> adder_tree1/1(sync)
